simulink model "Power_Model"  (R2018a)
settings: Solver=FixedStepDiscrete  StartTime=0.0  StopTime=10.0  FixedStep=1e-6  RelTol=1e-3
undefined symbols (not defined in the file or in its folder): Ion, Lithium
libraries: powerlib x14, powerlib_meascontrol x2, electricdrivelib x1, re_lib x1
settings Model: Creator=User  LastModifiedBy=User

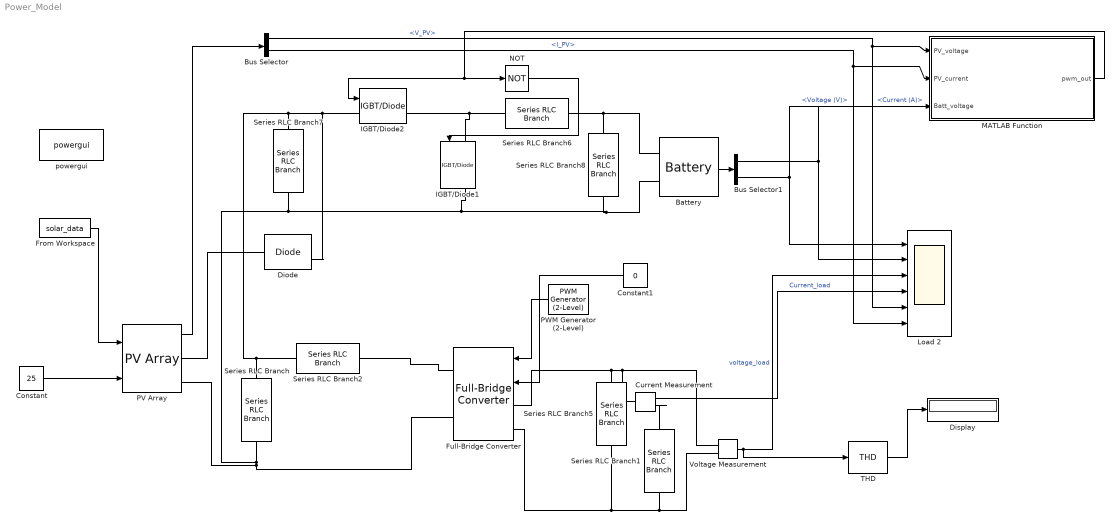
== system Power_Model ==
  Battery : electricdrivelib/Extra Sources/Battery  BatType=Lithium-Ion  ShowTempParam=off  ThermalPreset=no  ShowAgeParam=off  NomV=24  NomQ=182.87  SOC=80  Batt_Tr=30  PresetModel=off  MaxQ=182.87  MinV=21  FullV=29.4  Dis_rate=91.4  R=0.02  Normal_OP=182.87  expZone="[26.5      200]"  current=[6.5 13 32.5]  Units=Time  Tci=20  NomT=20  T2=-30  MaxQ2=4.8  FullV2=7.1  Normal_OP2=5.655  expZone2="[6.58           1]"  Rca=0.6  ti=2000  Dp=0  Neq0=0  Tsim=1e6  Ta1=25  Qeol=5.4*0.9  Reol=0.013333*1.2  Char_age=[2.3478, 3]  Dis_age=[2.3478, 10]  N1=1500  N2=10500  N3=1000  N4=1400  Ta2=45  N5=950
  Bus Selector : BusSelector  OutputSignals=V_PV,I_PV
  Bus Selector1 : BusSelector  OutputSignals=Current (A),Voltage (V)
  Constant : Constant  Value=25
  Constant1 : Constant  Value=0
  Current Measurement : powerlib/Measurements/Current Measurement  PhasorSimulation=off  OutputType=Complex  PSBequivalent=0
  Diode : powerlib/Power Electronics/Diode  Ron=0.001  Lon=0  Vf=0.8  IC=0  UseSnubber=0  Rs=500  Cs=250e-9  Measurements=on
  Display : Display
  From Workspace : FromWorkspace  VariableName=solar_data  SampleTime=0
  Full-Bridge Converter : powerlib/Power Electronics/Full-Bridge Converter  ModelType=Switching devices  Ron=1e-3  Rs=1e6  Cs=inf  Vforward=[0,0]  Ron_Diode=1e-3  Rs_Diode=1e6  Cs_Diode=inf  Vf_Diode=1e-3  Rs_CurrentSource=inf
      settings: SourceProductName=Simscape Power Systems  SourceProductBaseCode=PS
  IGBT/Diode1 : powerlib/Power Electronics/IGBT//Diode  Ron=1e-3  Rs=1e5  Cs=inf  Measurements=on
  IGBT/Diode2 : powerlib/Power Electronics/IGBT//Diode  Ron=1e-3  Rs=1e5  Cs=inf  Measurements=on
  Load 2 : Scope  NumInputPorts=6
  MATLAB Function : MATLAB Function  TreatAsAtomicUnit=on
  NOT : Logic  Operator=NOT  IconShape=distinctive  AllPortsSameDT=off  OutDataTypeStr=boolean
  PV Array : re_lib/Solar/PV Array  Npar=2  Nser=6  PlotType=array @ 25 deg.C & specified irradiances  S_vec="[ 300  200  100 ]"  Temp_C_vec="[ 25 85  ]"  ModuleName=User-defined  PlotWhenSelected=off  Pm=595.7965  Ncell=78  Voc=55.02  Isc=13.67  Vm=46.15  Im=12.91  beta_Voc_pc=-0.27  alpha_Isc_pc=0.04  beta_Voc=-0.14855  alpha_Isc=0.005468  IL=13.6808  I0=1.2384e-11  nI=0.99063  Rsh=257.239  Rs=0.20377  BAL=off  Tc=1e-6  Tfilter=5e-5
  PWM Generator (2-Level) : powerlib_meascontrol/Pulse & Signal Generators/PWM Generator (2-Level)  ModulatorType=Single-phase full-bridge (4 pulses)  ModulatorMode=Unsynchronized  Fc=10000  Pc=90  nF=27  MinMax=[ -1 1]  SamplingTechnique=Symmetrical regular (single edge)  ModulatingSignals=on  m=1  Freq=50  Phase=0  Ts=5e-6  ShowCarrierOutport=off
      settings: SourceProductName=Simscape Power Systems
  Series RLC Branch : powerlib/Elements/Series RLC Branch  LConnTagsString=__new0  RConnTagsString=__new0  BranchType=C  Resistance=1  Inductance=1e-3  SetiL0=off  InitialCurrent=0  Capacitance=1e-6  Setx0=off  InitialVoltage=0  Measurements=None
  Series RLC Branch1 : powerlib/Elements/Series RLC Branch  LConnTagsString=__new0  RConnTagsString=__new0  BranchType=RL  Resistance=1000  Inductance=0.174  SetiL0=off  InitialCurrent=0  Capacitance=1e-6  Setx0=off  InitialVoltage=0  Measurements=None
  Series RLC Branch2 : powerlib/Elements/Series RLC Branch  LConnTagsString=__new0  RConnTagsString=__new0  BranchType=L  Resistance=1  Inductance=1e-3  SetiL0=off  InitialCurrent=0  Capacitance=1e-6  Setx0=off  InitialVoltage=0  Measurements=None
  Series RLC Branch5 : powerlib/Elements/Series RLC Branch  LConnTagsString=__new0  RConnTagsString=__new0  BranchType=C  Resistance=1  Inductance=1e-3  SetiL0=off  InitialCurrent=0  Capacitance=30e-6  Setx0=off  InitialVoltage=0  Measurements=None
  Series RLC Branch6 : powerlib/Elements/Series RLC Branch  LConnTagsString=__new0  RConnTagsString=__new0  BranchType=RL  Resistance=1  Inductance=1e-3  SetiL0=off  InitialCurrent=0  Capacitance=1e-6  Setx0=off  InitialVoltage=0  Measurements=None
  Series RLC Branch7 : powerlib/Elements/Series RLC Branch  LConnTagsString=__new0  RConnTagsString=__new0  BranchType=RC  Resistance=1  Inductance=1e-3  SetiL0=off  InitialCurrent=0  Capacitance=1e-6  Setx0=off  InitialVoltage=0  Measurements=None
  Series RLC Branch8 : powerlib/Elements/Series RLC Branch  LConnTagsString=__new0  RConnTagsString=__new0  BranchType=C  Resistance=1  Inductance=1e-3  SetiL0=off  InitialCurrent=0  Capacitance=1e-6  Setx0=off  InitialVoltage=0  Measurements=None
  THD : powerlib_meascontrol/Measurements/THD  Freq=50  Ts=5e-5
  Voltage Measurement : powerlib/Measurements/Voltage Measurement  PhasorSimulation=off  OutputType=Complex  PSBequivalent=0
  powergui : powerlib/powergui  Priority=1  SimulationMode=Discrete  SampleTime=5e-5  frequency=60  Iterations=50  frequencyindice=0  Pbase=100e6  ErrMax=1e-4  UnitsV=kV  UnitsW=MW  buscounter=0  FunctionMessages=off  echomessages=off  EnableUseOfTLC=off  CurrentSourceSwitches=off  DisableSnubberDevices=off  DisableRonSwitches=off  DisableVfSwitches=off  DisplayEquations=off  SolverType=Tustin/Backward Euler (TBE)  Interpol=off  ExternalGateDelay=off  methode=off  Ts=100  x0status=blocks  SPID=off  SwTol=0  HookPort=off  RestoreLinks=warning  ResistiveCurrentMeasurement=off  Frange=[0:2:500]  Ylog=off  Xlog=on  ShowGrid=off  save=off  variable=ZData  structure=0  ZoomFFT=off  StartTime=0.0  cycles=1  DisplayStyle=1  fundamental=60  FreqAxis=off  MaxFrequency=1000  frequencyindicesteady=1  RmsSteady=1  display=off
  wires:
  Battery/1 -> Bus Selector1/1
  Bus Selector/2 -> Load 2/6, MATLAB Function/2(PV_current)  "<I_PV>"
  Bus Selector1/1 -> Load 2/2  "<Current (A)>"
  THD/1 -> Display/1
  From Workspace/1 -> PV Array/1
  PV Array/1 -> Bus Selector/1
  Bus Selector/1 -> Load 2/5, MATLAB Function/1(PV_voltage)  "<V_PV>"
  Voltage Measurement/1 -> THD/1, Load 2/3  "voltage_load"
  Current Measurement/1 -> Load 2/4  "Current_load"
  PWM Generator (2-Level)/1 -> Full-Bridge Converter/1
  Bus Selector1/2 -> Load 2/1, MATLAB Function/3(Batt_voltage)  "<Voltage (V)>"
  MATLAB Function/1(pwm_out) -> NOT/1, IGBT/Diode2/1
  Constant1/1 -> Full-Bridge Converter/2
  Constant/1 -> PV Array/2
  NOT/1 -> IGBT/Diode1/1
  connections:
  Current Measurement/LConn1 -- Series RLC Branch5/LConn1 -- Full-Bridge Converter/LConn1 -- Voltage Measurement/LConn1
  Series RLC Branch7/RConn1 -- IGBT/Diode1/RConn1 -- Series RLC Branch8/RConn1 -- Battery/LConn2 -- PV Array/RConn2 -- Full-Bridge Converter/RConn2 -- Series RLC Branch/RConn1
  Series RLC Branch6/RConn1 -- Series RLC Branch8/LConn1 -- Battery/LConn1
  Series RLC Branch6/LConn1 -- IGBT/Diode2/RConn1 -- IGBT/Diode1/LConn1
  Series RLC Branch7/LConn1 -- IGBT/Diode2/LConn1 -- Diode/RConn1 -- Series RLC Branch2/LConn1 -- Series RLC Branch/LConn1
  Voltage Measurement/LConn2 -- Series RLC Branch1/RConn1 -- Full-Bridge Converter/LConn2 -- Series RLC Branch5/RConn1
  Current Measurement/RConn1 -- Series RLC Branch1/LConn1
  Series RLC Branch2/RConn1 -- Full-Bridge Converter/RConn1
  Diode/LConn1 -- PV Array/RConn1

== matlab function Power_Model/MATLAB Function ==
  settings: updateMethod=DISCRETE
  data: PV_voltage input; pwm_out output; PV_current input; Batt_voltage input
function pwm_out = PSO_MPPCharging(PV_voltage, PV_current, Batt_voltage)
    % Persistent variables to retain values across function calls
    persistent prev_error prev_pwm

    if isempty(prev_error)
        prev_error = 0;       % Initialize prev_error if it's the first call
    end
    if isempty(prev_pwm)
        prev_pwm = 0.5;       % Initialize prev_pwm if it's the first call
    end

    % Constants 
    Vpv_ref = 25.9;  
    Vdc_min = 21;  
    Vdc_max = 29.4; 

    % Calculate the current power of the PV array
    pv_power = PV_voltage * PV_current;
    
    % Calculate the current error (Power deviation) for MPPT
    error = pv_power - (prev_pwm * Vpv_ref);  % Error between current and previous PWM output
    
    % Perturb and Observe algorithm
    if error > prev_error
        perturb = 1;  % Increase the duty cycle for MPPT
    elseif error < prev_error
        perturb = -1; % Decrease the duty cycle for MPPT
    else
        perturb = 0;  % No change
    end

    % Calculate the PWM duty cycle for PV
    delta_pwm = perturb * 0.1;  % Adjust step size for MPPT
    pwm_duty = prev_pwm + delta_pwm;
    
    % Keep the PWM duty within safe bounds (0-1 range)
    pwm_duty = min(max(pwm_duty, 0), 1);
    
    % Charging control for the battery based on its voltage
    if Batt_voltage < Vdc_min
        pwm_out = pwm_duty + 0.1;
    elseif Batt_voltage > Vdc_max
        pwm_out = pwm_duty - 0.1;
    else
        pwm_out = pwm_duty;
    end

    % Ensure the PWM duty
    pwm_out = min(max(pwm_out, 0), 1);
    
    % Update previous error and PWM for next iteration
    prev_error = error;  % Update the previous error
    prev_pwm = pwm_out;  % Update the previous PWM for next step
end
